simulink model "KFPIDtest2"  (R2015a)
settings: Solver=ode5  StartTime=0.0  StopTime=100  FixedStep=0.01  RelTol=1e-3
libraries: simulink x2
settings Model: Creator=LAB425  LastModifiedBy=LAB425

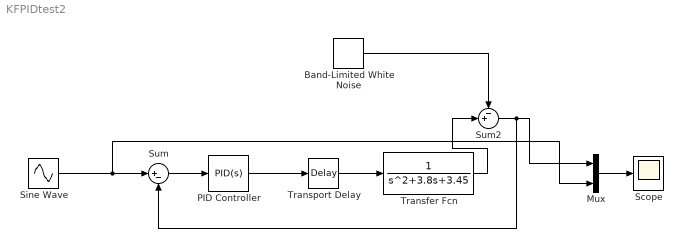
== system KFPIDtest2 ==
  Band-Limited White Noise : simulink/Sources/Band-Limited White Noise  Cov=[0.00001]  Ts=0.01  seed=[23341]
  Mux : Mux  Inputs=2
  PID Controller : simulink/Continuous/PID Controller  Controller=PID  TimeDomain=Continuous-time  SampleTime=-1  IntegratorMethod=Forward Euler  FilterMethod=Forward Euler  Form=Parallel  UseFilter=on  ControllerParametersSource=internal  P=60  I=4  D=0  N=100  InitialConditionSource=internal  InitialConditionForIntegrator=0  InitialConditionForFilter=0  ExternalReset=none  LimitOutput=off  UpperSaturationLimit=inf  LowerSaturationLimit=-inf  LinearizeAsGain=on  AntiWindupMode=none  Kb=1  TrackingMode=off  Kt=1  PParamMin=[]  PParamMax=[]  IParamMin=[]  IParamMax=[]  DParamMin=[]  DParamMax=[]  NParamMin=[]  NParamMax=[]  KbParamMin=[]  KbParamMax=[]  KtParamMin=[]  KtParamMax=[]  POutMin=[]  POutMax=[]  IOutMin=[]  IOutMax=[]  DOutMin=[]  DOutMax=[]  NOutMin=[]  NOutMax=[]  KbOutMin=[]  KbOutMax=[]  KtOutMin=[]  KtOutMax=[]  IntegratorOutMin=[]  IntegratorOutMax=[]  FilterOutMin=[]  FilterOutMax=[]  SumOutMin=[]  SumOutMax=[]  SumI1OutMin=[]  SumI1OutMax=[]  SumI2OutMin=[]  SumI2OutMax=[]  SumI3OutMin=[]  SumI3OutMax=[]  SumDOutMin=[]  SumDOutMax=[]  SaturationOutMin=[]  SaturationOutMax=[]  IntegratorContinuousStateAttributes=''  IntegratorStateMustResolveToSignalObject=off  IntegratorRTWStateStorageClass=Auto  FilterContinuousStateAttributes=''  FilterStateMustResolveToSignalObject=off  FilterRTWStateStorageClass=Auto  DifferentiatorICPrevScaledInput=0  DifferentiatorOutMin=[]  DifferentiatorOutMax=[]
  Scope : Scope
      settings: TimeRange=10  YMin=-25000000  YMax=10000000
  Sine Wave : Sin  Amplitude=1.95  SampleTime=0
  Sum : Sum  Inputs=|+-
  Sum2 : Sum  Inputs=-+|
  Transfer Fcn : TransferFcn  Denominator=[1 3.8 3.45]
  Transport Delay : TransportDelay  DelayTime=0.05
  wires:
  Sum/1 -> PID Controller/1
  Sine Wave/1 -> Mux/2, Sum/1
  Mux/1 -> Scope/1
  PID Controller/1 -> Transport Delay/1
  Transport Delay/1 -> Transfer Fcn/1
  Transfer Fcn/1 -> Sum2/2
  Band-Limited White Noise/1 -> Sum2/1
  Sum2/1 -> Sum/2, Mux/1
